simulink model "comHost"  (R2020b)
settings: Solver=VariableStepAuto  StartTime=0.0  StopTime=30  RelTol=1e-3
undefined symbols (not defined in the file or in its folder): f
libraries: parrotlib x1, instrumentlib x1
settings Model: Creator=USER  LastModifiedBy=USER

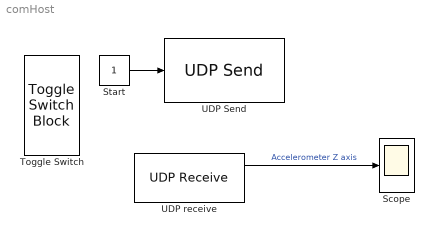
== system comHost ==
  Scope : Scope
  "Start " : Constant  OutDataTypeStr=single  SampleTime=0.05
  Toggle Switch : ToggleSwitchBlock
      settings: Values={{'Off', 'On'}, [0 1]}
  UDP Send : parrotlib/UDP Send  remoteURL='192.168.3.1'  remotePort=29000  localURL='0.0.0.0'  localPortSource=Automatically determine  localPort=2048  sendBufferSize=8192  sampletime=-1  blockPlatform=LINUX  separateLengthPort=0
      settings: SourceProductBaseCode=MINIDRONES
  UDP receive : instrumentlib/UDP Receive  Host=192.168.3.1  Port=25000  LocalPort=25000  EnablePortSharing=off  GetLatestData=off  DataSize=1  DataType=double  ASCIIFormatting=%f,  Terminator=LF  ByteOrder=LittleEndian  EnableBlockingMode=off  Timeout=10  SampleTime=1  LocalAddress=192.168.3.2
      settings: SourceProductName=Instrument Control Toolbox
  wires:
  "Start "/1 -> UDP Send/1
  UDP receive/1 -> Scope/1  "Accelerometer Z axis"
